simulink model "APID"  (R2021a)
settings: Solver=VariableStepAuto  StartTime=0.0  StopTime=100  RelTol=1e-6  AbsTol=1e-6
undefined symbols (not defined in the file or in its folder): DiscIntNeverNeededParam, G, k, Solar_time, wind, wind_time
libraries: powerlib_extras x24, simulink x2
(part 1 of 2)
settings Model: Creator=hp  LastModifiedBy=hp
settings SolverCC: ZeroCrossAlgorithm=Adaptive
settings DataIOCC: ReturnWorkspaceOutputs=off
settings DebuggingCC: MaskedZcDiagnostic=none  IgnoredZcDiagnostic=none

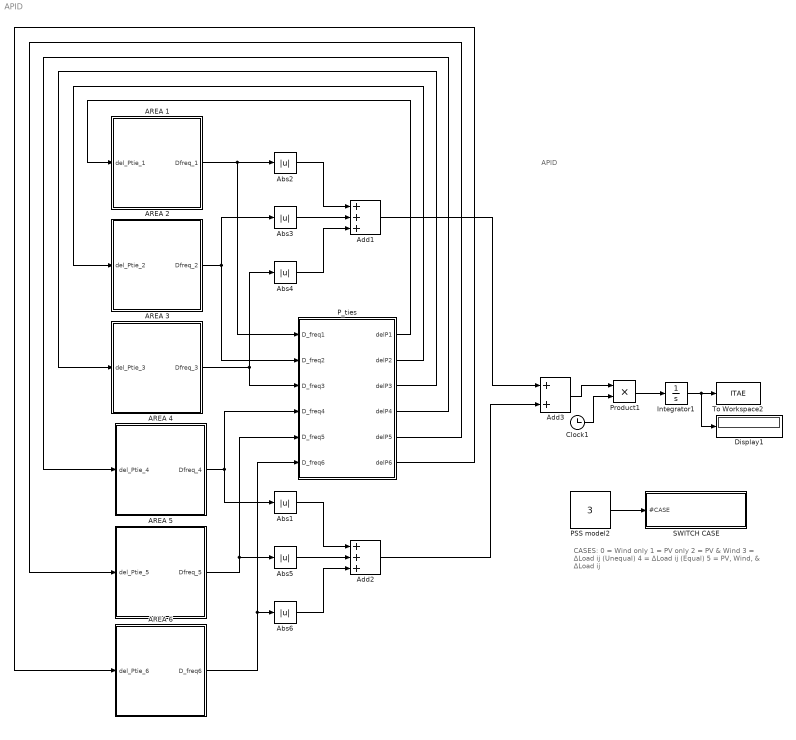
== system APID ==
  note: APID
  note: CASES:
      |
      | 0 = Wind only
      | 1 = PV only
      | 2 = PV & Wind
      | 3 = ΔLoad ij (Unequal)
      | 4 = ΔLoad ij (Equal)
      | 5 = PV, Wind, & ΔLoad ij
  AREA 1 : Subsystem
  AREA 2 : Subsystem
  AREA 3 : Subsystem
  AREA 4 : Subsystem
  AREA 5 : Subsystem
  AREA 6 : Subsystem
  Abs{1..6} (6 alike) : Abs
  Add1 : Sum  Inputs=+++
  Add2 : Sum  Inputs=+++
  Add3 : Sum
  Clock1 : Clock
  Display1 : Display
  Integrator1 : Integrator
  PSS model2 : Constant  Value=3
  P_ties : Subsystem
  Product1 : Product
  SWITCH CASE : Subsystem
  To Workspace2 : ToWorkspace  VariableName=ITAE  SampleTime=-1
      settings: Save2DSignal=2-D array (concatenate along first dimension)
  wires:
  P_ties/1(delP1) -> AREA 1/1(del_Ptie_1)
  Abs2/1 -> Add1/1
  AREA 1/1(Dfreq_1) -> P_ties/1(D_freq1), Abs2/1
  Abs4/1 -> Add1/3
  Abs3/1 -> Add1/2
  P_ties/5(delP5) -> AREA 5/1(del_Ptie_5)
  P_ties/4(delP4) -> AREA 4/1(del_Ptie_4)
  Clock1/1 -> Product1/2
  P_ties/6(delP6) -> AREA 6/1(del_Ptie_6)
  P_ties/2(delP2) -> AREA 2/1(del_Ptie_2)
  AREA 3/1(Dfreq_3) -> P_ties/3(D_freq3), Abs4/1
  Product1/1 -> Integrator1/1
  AREA 2/1("Dfreq_2   ") -> P_ties/2(D_freq2), Abs3/1
  Integrator1/1 -> To Workspace2/1, Display1/1
  P_ties/3(delP3) -> AREA 3/1(del_Ptie_3)
  Abs5/1 -> Add2/2
  Abs6/1 -> Add2/3
  Abs1/1 -> Add2/1
  AREA 4/1(Dfreq_4) -> Abs1/1, P_ties/4(D_freq4)
  AREA 5/1(Dfreq_5) -> P_ties/5(D_freq5), Abs5/1
  AREA 6/1(D_freq6) -> P_ties/6(D_freq6), Abs6/1
  Add3/1 -> Product1/1
  Add1/1 -> Add3/1
  Add2/1 -> Add3/2
  PSS model2/1 -> SWITCH CASE/1(#CASE)

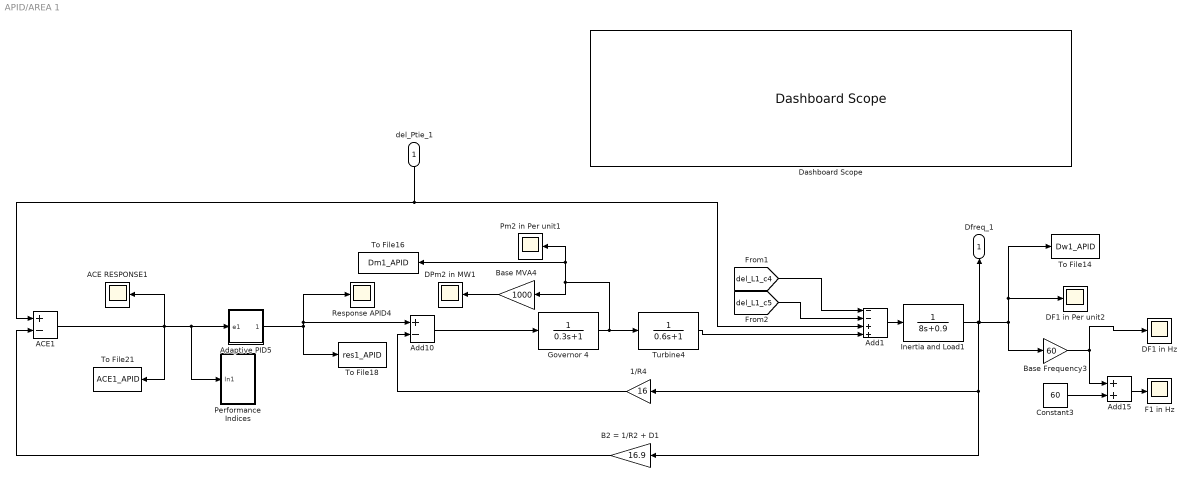
== system APID/AREA 1 ==
  del_Ptie_1 : Inport
  1/R4 : Gain  Gain=16
  ACE RESPONSE1 : Scope
  ACE1 : Sum  Inputs=+-
  Adaptive PID5 : Subsystem  mask{gamma=k}
  Add1 : Sum  Inputs=--++
  Add10 : Sum  Inputs=+-
  Add15 : Sum
  B2 = 1/R2 + D1 : Gain  Gain=16.9
  Base Frequency3 : Gain  Gain=60
  Base MVA4 : Gain  Gain=1000
  Constant3 : Constant  Value=60
  DF1 in Hz : Scope
  DF1 in Per unit2 : Scope
  DPm2 in MW1 : Scope
  Dashboard Scope : DashboardScope
  F1 in Hz : Scope
  Governor 4 : TransferFcn  Denominator=[0.3 1]
  Inertia and Load1 : TransferFcn  Denominator=[8 0.9]
  Performance Indices : Subsystem
  Pm2 in Per unit1 : Scope
  Response APID4 : Scope
  To File14 : ToFile  Filename=Dw1_APID  MatrixName=Dw1_APID
  To File16 : ToFile  Filename=Dm1_APID  MatrixName=Dm1_APID
  To File18 : ToFile  Filename=res1_APID  MatrixName=res1_APID
  To File21 : ToFile  Filename=ACE1_APID  MatrixName=ACE1_APID
  Turbine4 : TransferFcn  Denominator=[0.6 1]
  Dfreq_1 : Outport
  wires:
  Base Frequency3/1 -> DF1 in Hz/1, Add15/1
  Add1/1 -> Inertia and Load1/1
  1/R4/1 -> Add10/2
  Add15/1 -> F1 in Hz/1
  B2 = 1/R2 + D1/1 -> ACE1/2
  Governor 4/1 -> To File16/1, Pm2 in Per unit1/1, Base MVA4/1, Turbine4/1
  Inertia and Load1/1 -> Base Frequency3/1, To File14/1, DF1 in Per unit2/1, Dfreq_1/1, 1/R4/1, B2 = 1/R2 + D1/1
  Base MVA4/1 -> DPm2 in MW1/1
  ACE1/1 -> Adaptive PID5/1(e1), Performance Indices/1(In1), To File21/1, ACE RESPONSE1/1
  Adaptive PID5/1(u(t)) -> Response APID4/1, Add10/1, To File18/1
  Constant3/1 -> Add15/2
  Add10/1 -> Governor 4/1
  [del_L1_c5] -> Add1/2
  Turbine4/1 -> Add1/4
  del_Ptie_1/1 -> ACE1/1, Add1/3
  [del_L1_c4] -> Add1/1

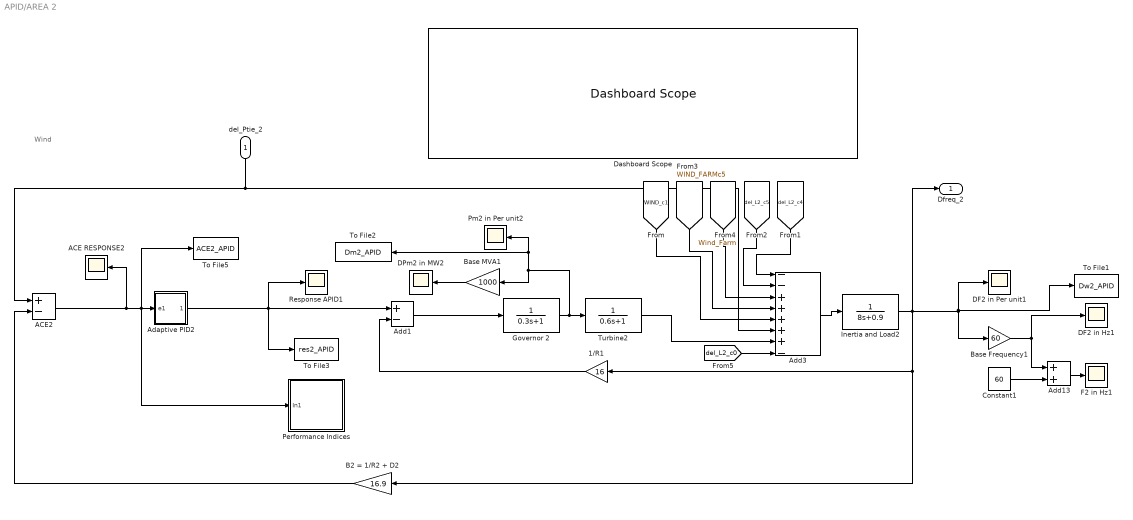
== system APID/AREA 2 ==
  note: Wind
  del_Ptie_2 : Inport
  1/R1 : Gain  Gain=16
  ACE RESPONSE2 : Scope
  ACE2 : Sum  Inputs=+-
  Adaptive PID2 : Subsystem  mask{gamma=k}
  Add1 : Sum  Inputs=+-
  Add13 : Sum
  Add3 : Sum  Inputs=--+++++-
  B2 = 1/R2 + D2 : Gain  Gain=16.9
  Base Frequency1 : Gain  Gain=60
  Base MVA1 : Gain  Gain=1000
  Constant1 : Constant  Value=60
  DF2 in Hz1 : Scope
  DF2 in Per unit1 : Scope
  DPm2 in MW2 : Scope
  Dashboard Scope : DashboardScope
  F2 in Hz1 : Scope
  Governor 2 : TransferFcn  Denominator=[0.3 1]
  Inertia and Load2 : TransferFcn  Denominator=[8 0.9]
  Performance Indices : Subsystem
  Pm2 in Per unit2 : Scope
  Response APID1 : Scope
  To File1 : ToFile  Filename=Dw2_APID  MatrixName=Dw2_APID
  To File2 : ToFile  Filename=Dm2_APID  MatrixName=Dm2_APID
  To File3 : ToFile  Filename=res2_APID  MatrixName=res2_APID
  To File5 : ToFile  Filename=ACE2_APID  MatrixName=ACE2_APID
  Turbine2 : TransferFcn  Denominator=[0.6 1]
  "Dfreq_2   " : Outport
  wires:
  Add13/1 -> F2 in Hz1/1
  1/R1/1 -> Add1/2
  Base Frequency1/1 -> Add13/1, DF2 in Hz1/1
  Constant1/1 -> Add13/2
  Governor 2/1 -> Turbine2/1, Base MVA1/1, To File2/1, Pm2 in Per unit2/1
  Add3/1 -> Inertia and Load2/1
  B2 = 1/R2 + D2/1 -> ACE2/2
  Inertia and Load2/1 -> 1/R1/1, B2 = 1/R2 + D2/1, "Dfreq_2   "/1, DF2 in Per unit1/1, To File1/1, Base Frequency1/1
  Base MVA1/1 -> DPm2 in MW2/1
  ACE2/1 -> Performance Indices/1(In1), Adaptive PID2/1(e1), To File5/1, ACE RESPONSE2/1
  Add1/1 -> Governor 2/1
  Adaptive PID2/1(u(t)) -> Add1/1, Response APID1/1, To File3/1
  Turbine2/1 -> Add3/7
  [del_L2_c5] -> Add3/2
  del_Ptie_2/1 -> Add3/6, ACE2/1
  [WIND_FARMc5] -> Add3/4
  [WIND_c1] -> Add3/5
  [Wind_Farm] -> Add3/3
  [del_L2_c4] -> Add3/1
  [del_L2_c0] -> Add3/8

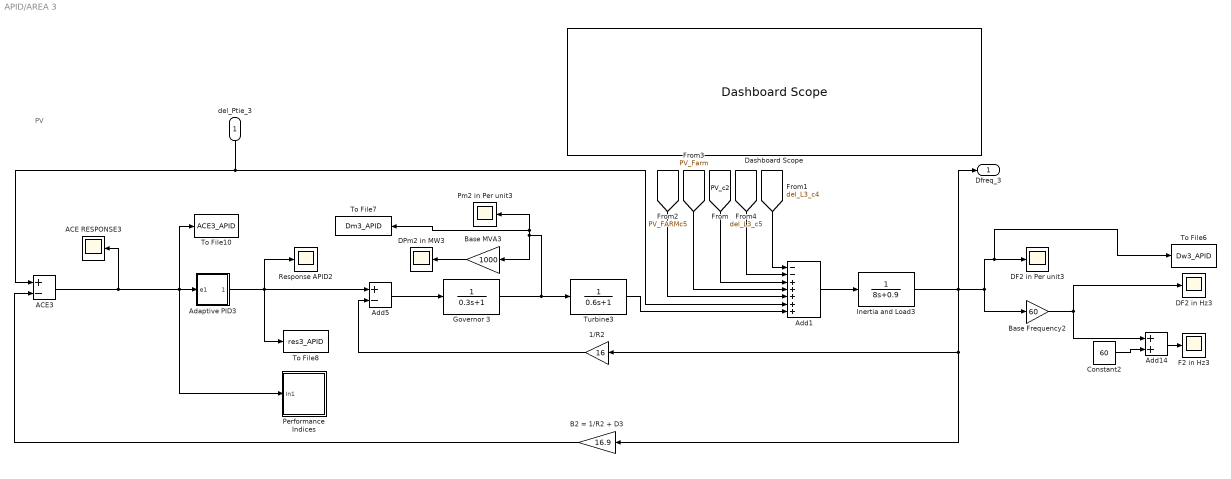
== system APID/AREA 3 ==
  note: PV
  del_Ptie_3 : Inport
  1/R2 : Gain  Gain=16
  ACE RESPONSE3 : Scope
  ACE3 : Sum  Inputs=+-
  Adaptive PID3 : Subsystem  mask{gamma=k}
  Add1 : Sum  Inputs=--+++++
  Add14 : Sum
  Add5 : Sum  Inputs=+-
  B2 = 1/R2 + D3 : Gain  Gain=16.9
  Base Frequency2 : Gain  Gain=60
  Base MVA3 : Gain  Gain=1000
  Constant2 : Constant  Value=60
  DF2 in Hz3 : Scope
  DF2 in Per unit3 : Scope
  DPm2 in MW3 : Scope
  Dashboard Scope : DashboardScope
  F2 in Hz3 : Scope
  Governor 3 : TransferFcn  Denominator=[0.3 1]
  Inertia and Load3 : TransferFcn  Denominator=[8 0.9]
  Performance Indices : Subsystem
  Pm2 in Per unit3 : Scope
  Response APID2 : Scope
  To File10 : ToFile  Filename=ACE3_APID  MatrixName=ACE3_APID
  To File6 : ToFile  Filename=Dw3_APID  MatrixName=Dw3_APID
  To File7 : ToFile  Filename=Dm3_APID  MatrixName=Dm3_APID
  To File8 : ToFile  Filename=res3_APID  MatrixName=res3_APID
  Turbine3 : TransferFcn  Denominator=[0.6 1]
  Dfreq_3 : Outport
  wires:
  Constant2/1 -> Add14/2
  Base MVA3/1 -> DPm2 in MW3/1
  Base Frequency2/1 -> Add14/1, DF2 in Hz3/1
  B2 = 1/R2 + D3/1 -> ACE3/2
  Add1/1 -> Inertia and Load3/1
  Add14/1 -> F2 in Hz3/1
  1/R2/1 -> Add5/2
  Governor 3/1 -> Turbine3/1, Base MVA3/1, To File7/1, Pm2 in Per unit3/1
  ACE3/1 -> Performance Indices/1(In1), To File10/1, Adaptive PID3/1(e1), ACE RESPONSE3/1
  Adaptive PID3/1(u(t)) -> Response APID2/1, Add5/1, To File8/1
  Add5/1 -> Governor 3/1
  Inertia and Load3/1 -> Dfreq_3/1, Base Frequency2/1, To File6/1, DF2 in Per unit3/1, B2 = 1/R2 + D3/1, 1/R2/1
  [PV_FARMc5] -> Add1/5
  Turbine3/1 -> Add1/7
  [del_L3_c5] -> Add1/2
  [del_L3_c4] -> Add1/1
  del_Ptie_3/1 -> Add1/6, ACE3/1
  [PV_c2] -> Add1/3
  [PV_Farm] -> Add1/4

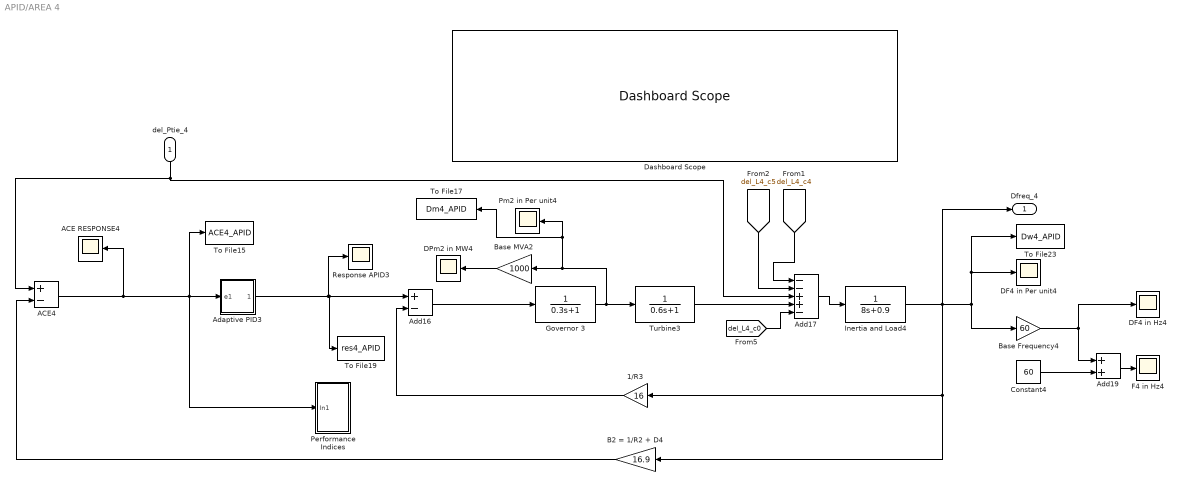
== system APID/AREA 4 ==
  del_Ptie_4 : Inport
  1/R3 : Gain  Gain=16
  ACE RESPONSE4 : Scope
  ACE4 : Sum  Inputs=+-
  Adaptive PID3 : Subsystem  mask{gamma=k}
  Add16 : Sum  Inputs=+-
  Add17 : Sum  Inputs=--++-
  Add19 : Sum
  B2 = 1/R2 + D4 : Gain  Gain=16.9
  Base Frequency4 : Gain  Gain=60
  Base MVA2 : Gain  Gain=1000
  Constant4 : Constant  Value=60
  DF4 in Hz4 : Scope
  DF4 in Per unit4 : Scope
  DPm2 in MW4 : Scope
  Dashboard Scope : DashboardScope
  F4 in Hz4 : Scope
  Governor 3 : TransferFcn  Denominator=[0.3 1]
  Inertia and Load4 : TransferFcn  Denominator=[8 0.9]
  Performance Indices : Subsystem
  Pm2 in Per unit4 : Scope
  Response APID3 : Scope
  To File15 : ToFile  Filename=ACE4_APID  MatrixName=ACE4_APID
  To File17 : ToFile  Filename=Dm4_APID  MatrixName=Dm4_APID
  To File19 : ToFile  Filename=res4_APID  MatrixName=res4_APID
  To File23 : ToFile  Filename=Dw4_APID  MatrixName=Dw4_APID
  Turbine3 : TransferFcn  Denominator=[0.6 1]
  Dfreq_4 : Outport
  wires:
  Add17/1 -> Inertia and Load4/1
  Add19/1 -> F4 in Hz4/1
  Constant4/1 -> Add19/2
  Governor 3/1 -> Turbine3/1, Base MVA2/1, To File17/1, Pm2 in Per unit4/1
  B2 = 1/R2 + D4/1 -> ACE4/2
  1/R3/1 -> Add16/2
  Inertia and Load4/1 -> Dfreq_4/1, To File23/1, DF4 in Per unit4/1, Base Frequency4/1, 1/R3/1, B2 = 1/R2 + D4/1
  Base Frequency4/1 -> Add19/1, DF4 in Hz4/1
  Base MVA2/1 -> DPm2 in MW4/1
  Add16/1 -> Governor 3/1
  ACE4/1 -> Adaptive PID3/1(e1), Performance Indices/1(In1), To File15/1, ACE RESPONSE4/1
  del_Ptie_4/1 -> Add17/3, ACE4/1
  Turbine3/1 -> Add17/4
  Adaptive PID3/1(u(t)) -> Response APID3/1, To File19/1, Add16/1
  [del_L4_c5] -> Add17/2
  [del_L4_c4] -> Add17/1
  [del_L4_c0] -> Add17/5

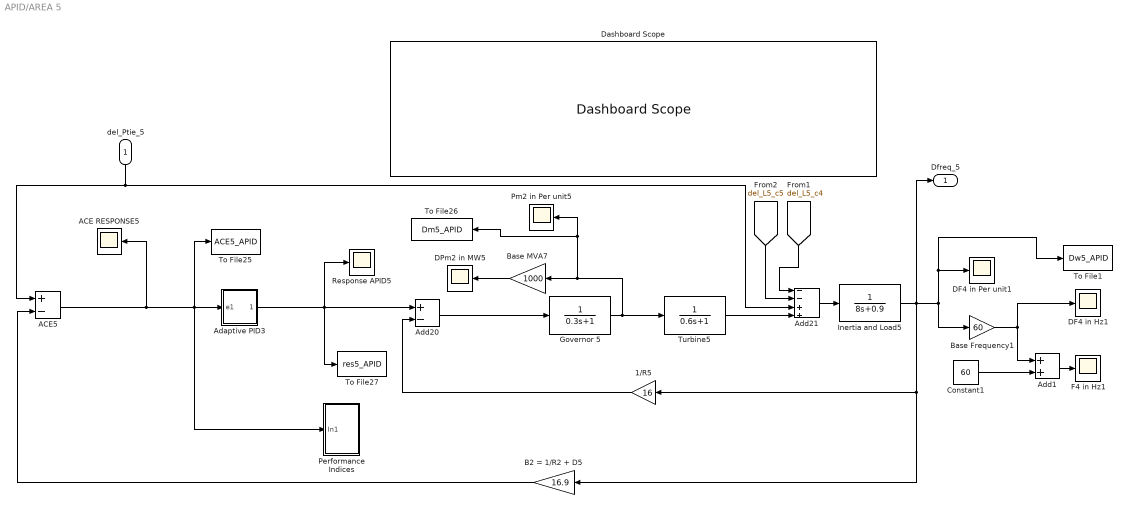
== system APID/AREA 5 ==
  del_Ptie_5 : Inport
  1/R5 : Gain  Gain=16
  ACE RESPONSE5 : Scope
  ACE5 : Sum  Inputs=+-
  Adaptive PID3 : Subsystem  mask{gamma=k}
  Add1 : Sum
  Add20 : Sum  Inputs=+-
  Add21 : Sum  Inputs=--++
  B2 = 1/R2 + D5 : Gain  Gain=16.9
  Base Frequency1 : Gain  Gain=60
  Base MVA7 : Gain  Gain=1000
  Constant1 : Constant  Value=60
  DF4 in Hz1 : Scope
  DF4 in Per unit1 : Scope
  DPm2 in MW5 : Scope
  Dashboard Scope : DashboardScope
  F4 in Hz1 : Scope
  Governor 5 : TransferFcn  Denominator=[0.3 1]
  Inertia and Load5 : TransferFcn  Denominator=[8 0.9]
  Performance Indices : Subsystem
  Pm2 in Per unit5 : Scope
  Response APID5 : Scope
  To File1 : ToFile  Filename=Dw5_APID  MatrixName=Dw5_APID
  To File25 : ToFile  Filename=ACE5_APID  MatrixName=ACE5_APID
  To File26 : ToFile  Filename=Dm5_APID  MatrixName=Dm5_APID
  To File27 : ToFile  Filename=res5_APID  MatrixName=res5_APID
  Turbine5 : TransferFcn  Denominator=[0.6 1]
  Dfreq_5 : Outport
  wires:
  Constant1/1 -> Add1/2
  Add1/1 -> F4 in Hz1/1
  Base Frequency1/1 -> Add1/1, DF4 in Hz1/1
  B2 = 1/R2 + D5/1 -> ACE5/2
  Governor 5/1 -> Turbine5/1, Base MVA7/1, To File26/1, Pm2 in Per unit5/1
  Base MVA7/1 -> DPm2 in MW5/1
  Add21/1 -> Inertia and Load5/1
  1/R5/1 -> Add20/2
  Inertia and Load5/1 -> B2 = 1/R2 + D5/1, 1/R5/1, Dfreq_5/1, Base Frequency1/1, To File1/1, DF4 in Per unit1/1
  ACE5/1 -> Performance Indices/1(In1), Adaptive PID3/1(e1), To File25/1, ACE RESPONSE5/1
  del_Ptie_5/1 -> Add21/3, ACE5/1
  Turbine5/1 -> Add21/4
  Add20/1 -> Governor 5/1
  Adaptive PID3/1(u(t)) -> To File27/1, Response APID5/1, Add20/1
  [del_L5_c5] -> Add21/2
  [del_L5_c4] -> Add21/1

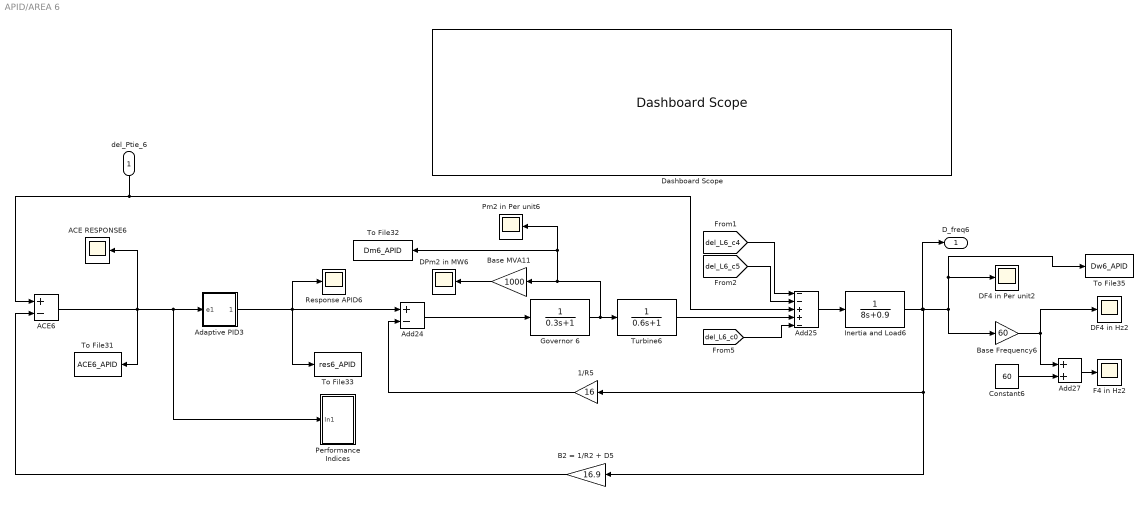
== system APID/AREA 6 ==
  del_Ptie_6 : Inport
  1/R5 : Gain  Gain=16
  ACE RESPONSE6 : Scope
  ACE6 : Sum  Inputs=+-
  Adaptive PID3 : Subsystem  mask{gamma=k}
  Add24 : Sum  Inputs=+-
  Add25 : Sum  Inputs=--++-
  Add27 : Sum
  B2 = 1/R2 + D5 : Gain  Gain=16.9
  Base Frequency6 : Gain  Gain=60
  Base MVA11 : Gain  Gain=1000
  Constant6 : Constant  Value=60
  DF4 in Hz2 : Scope
  DF4 in Per unit2 : Scope
  DPm2 in MW6 : Scope
  Dashboard Scope : DashboardScope
  F4 in Hz2 : Scope
  Governor 6 : TransferFcn  Denominator=[0.3 1]
  Inertia and Load6 : TransferFcn  Denominator=[8 0.9]
  Performance Indices : Subsystem
  Pm2 in Per unit6 : Scope
  Response APID6 : Scope
  To File31 : ToFile  Filename=ACE6_APID  MatrixName=ACE6_APID
  To File32 : ToFile  Filename=Dm6_APID  MatrixName=Dm6_APID
  To File33 : ToFile  Filename=res6_APID  MatrixName=res6_APID
  To File35 : ToFile  Filename=Dw6_APID  MatrixName=Dw6_APID
  Turbine6 : TransferFcn  Denominator=[0.6 1]
  D_freq6 : Outport
  wires:
  Constant6/1 -> Add27/2
  Base Frequency6/1 -> Add27/1, DF4 in Hz2/1
  Base MVA11/1 -> DPm2 in MW6/1
  Add27/1 -> F4 in Hz2/1
  Inertia and Load6/1 -> D_freq6/1, B2 = 1/R2 + D5/1, 1/R5/1, To File35/1, DF4 in Per unit2/1, Base Frequency6/1
  Governor 6/1 -> Turbine6/1, Base MVA11/1, Pm2 in Per unit6/1, To File32/1
  Add25/1 -> Inertia and Load6/1
  ACE6/1 -> To File31/1, Performance Indices/1(In1), Adaptive PID3/1(e1), ACE RESPONSE6/1
  Turbine6/1 -> Add25/4
  Add24/1 -> Governor 6/1
  Adaptive PID3/1(u(t)) -> To File33/1, Response APID6/1, Add24/1
  del_Ptie_6/1 -> Add25/3, ACE6/1
  1/R5/1 -> Add24/2
  B2 = 1/R2 + D5/1 -> ACE6/2
  [del_L6_c5] -> Add25/2
  [del_L6_c4] -> Add25/1
  [del_L6_c0] -> Add25/5

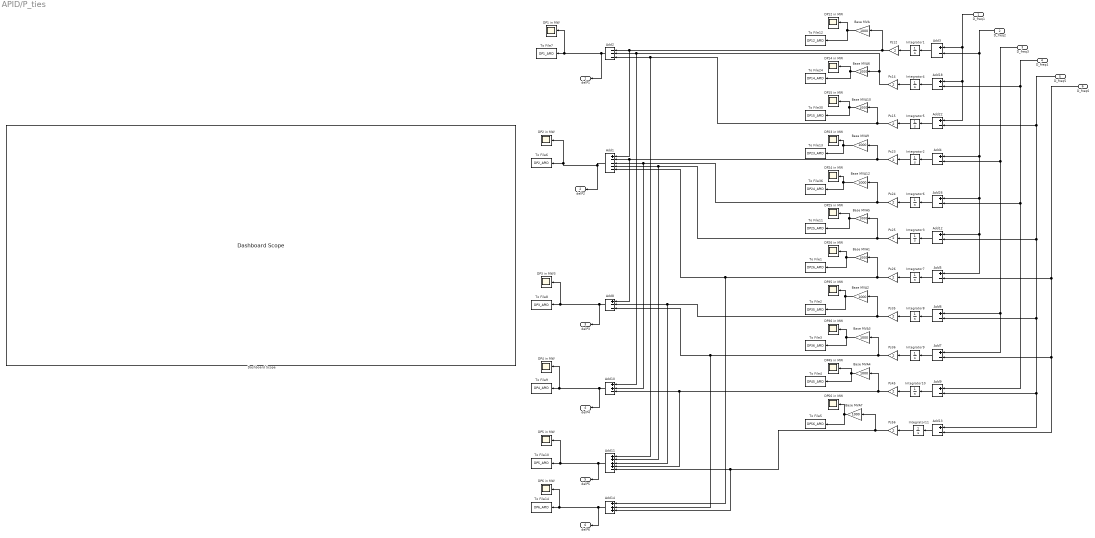
== system APID/P_ties ==
  D_freq1 : Inport
  D_freq2 : Inport  Port=2
  D_freq3 : Inport  Port=3
  D_freq4 : Inport  Port=4
  D_freq5 : Inport  Port=5
  D_freq6 : Inport  Port=6
  Add1 : Sum  Inputs=+----
  Add10 : Sum  Inputs=++-
  Add11 : Sum  Inputs=++++-
  Add{3..7,9,12..13,18,22,26} (11 alike) : Sum  Inputs=+-
  Add14 : Sum  Inputs=+++
  Add2 : Sum  Inputs=---
  Add8 : Sum  Inputs=+--
  Base MVA{,1..7,9..10,12} (11 alike) : Gain  Gain=1000
  DP1 in MW : Scope
  DP12 in MW : Scope
  DP14 in MW : Scope
  DP15 in MW : Scope
  DP2 in MW : Scope
  DP23 in MW : Scope
  DP24 in MW : Scope
  DP25 in MW : Scope
  DP26 in MW : Scope
  DP3 in MW3 : Scope
  DP35 in MW : Scope
  DP36 in MW : Scope
  DP4 in MW : Scope
  DP45 in MW : Scope
  DP5 in MW : Scope
  DP56 in MW : Scope
  DP6 in MW : Scope
  Dashboard Scope : DashboardScope
  Integrator{1..11} (11 alike) : Integrator
  Ps{12,14..15,23..26,35..36,45,56} (11 alike) : Gain  Gain=2
  To File1 : ToFile  Filename=DP26_APID  MatrixName=DP26_APID
  To File10 : ToFile  Filename=DP5_APID  MatrixName=DP5_APID
  To File11 : ToFile  Filename=DP25_APID  MatrixName=DP25_APID
  To File12 : ToFile  Filename=DP12_APID  MatrixName=DP12_APID
  To File13 : ToFile  Filename=DP23_APID  MatrixName=DP23_APID
  To File14 : ToFile  Filename=DP6_APID  MatrixName=DP6_APID
  To File2 : ToFile  Filename=DP35_APID  MatrixName=DP35_APID
  To File24 : ToFile  Filename=DP14_APID  MatrixName=DP14_APID
  To File3 : ToFile  Filename=DP36_APID  MatrixName=DP36_APID
  To File30 : ToFile  Filename=DP15_APID  MatrixName=DP15_APID
  To File36 : ToFile  Filename=DP24_APID  MatrixName=DP24_APID
  To File4 : ToFile  Filename=DP45_APID  MatrixName=DP45_APID
  To File5 : ToFile  Filename=DP56_APID  MatrixName=DP56_APID
  To File6 : ToFile  Filename=DP2_APID  MatrixName=DP2_APID
  To File7 : ToFile  Filename=DP1_APID  MatrixName=DP1_APID
  To File8 : ToFile  Filename=DP3_APID  MatrixName=DP3_APID
  To File9 : ToFile  Filename=DP4_APID  MatrixName=DP4_APID
  delP1 : Outport
  delP2 : Outport  Port=2
  delP3 : Outport  Port=3
  delP4 : Outport  Port=4
  delP5 : Outport  Port=5
  delP6 : Outport  Port=6
  wires:
  Ps12/1 -> Add1/1, Add2/1, Base MVA/1
  Add3/1 -> Integrator1/1
  Integrator1/1 -> Ps12/1
  Base MVA/1 -> To File12/1, DP12 in MW/1
  D_freq1/1 -> Add22/1, Add18/1, Add3/1
  D_freq2/1 -> Add5/1, Add12/1, Add26/1, Add4/1, Add3/2
  Ps14/1 -> Add10/1, Add2/2, Base MVA6/1
  Integrator4/1 -> Ps14/1
  Add18/1 -> Integrator4/1
  Base MVA6/1 -> To File24/1, DP14 in MW/1
  D_freq4/1 -> Add9/1, Add26/2, Add18/2
  Base MVA10/1 -> To File30/1, DP15 in MW/1
  Ps15/1 -> Add11/1, Add2/3, Base MVA10/1
  Integrator5/1 -> Ps15/1
  Add22/1 -> Integrator5/1
  D_freq5/1 -> Add9/2, Add13/1, Add6/2, Add12/2, Add22/2
  Integrator2/1 -> Ps23/1
  Add4/1 -> Integrator2/1
  Ps23/1 -> Base MVA9/1, Add8/1, Add1/2
  Base MVA9/1 -> DP23 in MW/1, To File13/1
  Base MVA12/1 -> DP24 in MW/1, To File36/1
  Integrator6/1 -> Ps24/1
  Ps24/1 -> Add10/2, Add1/3, Base MVA12/1
  Add26/1 -> Integrator6/1
  D_freq3/1 -> Add4/2, Add6/1, Add7/1
  Integrator3/1 -> Ps25/1
  Ps25/1 -> Add11/2, Add1/4, Base MVA5/1
  Base MVA5/1 -> To File11/1, DP25 in MW/1
  Add12/1 -> Integrator3/1
  Add5/1 -> Integrator7/1
  Base MVA1/1 -> To File1/1, DP26 in MW/1
  Integrator7/1 -> Ps26/1
  Ps26/1 -> Add14/1, Add1/5, Base MVA1/1
  D_freq6/1 -> Add5/2, Add7/2, Add13/2
  Base MVA2/1 -> To File2/1, DP35 in MW/1
  Ps35/1 -> Add11/3, Add8/2, Base MVA2/1
  Integrator8/1 -> Ps35/1
  Add6/1 -> Integrator8/1
  Add7/1 -> Integrator9/1
  Base MVA3/1 -> To File3/1, DP36 in MW/1
  Integrator9/1 -> Ps36/1
  Ps36/1 -> Add14/2, Add8/3, Base MVA3/1
  Ps45/1 -> Add11/4, Add10/3, Base MVA4/1
  Add9/1 -> Integrator10/1
  Integrator10/1 -> Ps45/1
  Base MVA4/1 -> DP45 in MW/1, To File4/1
  Integrator11/1 -> Ps56/1
  Add13/1 -> Integrator11/1
  Ps56/1 -> Add14/3, Add11/5, Base MVA7/1
  Base MVA7/1 -> DP56 in MW/1, To File5/1
  Add1/1 -> To File6/1, DP2 in MW/1, delP2/1
  Add2/1 -> DP1 in MW/1, To File7/1, delP1/1
  Add8/1 -> DP3 in MW3/1, To File8/1, delP3/1
  Add10/1 -> DP4 in MW/1, To File9/1, delP4/1
  Add11/1 -> DP5 in MW/1, To File10/1, delP5/1
  Add14/1 -> DP6 in MW/1, To File14/1, delP6/1

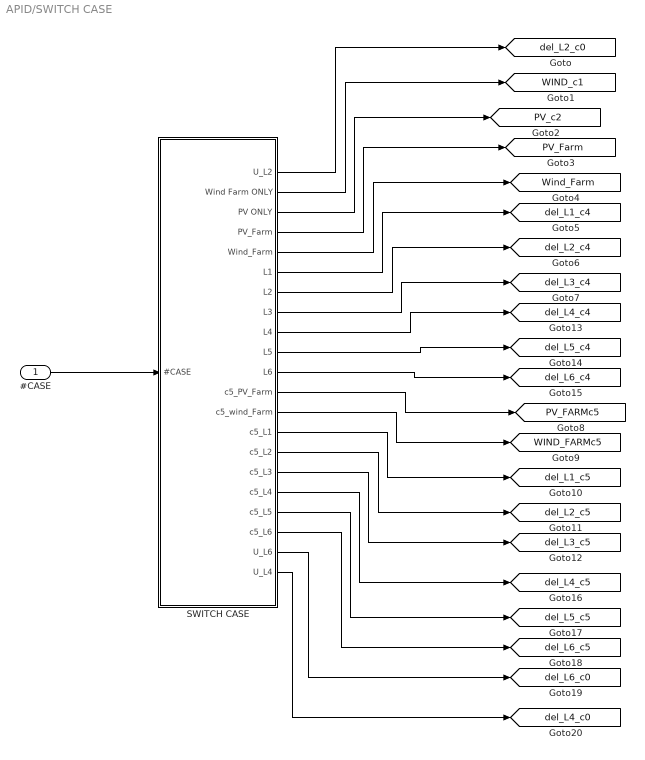
== system APID/SWITCH CASE ==
  #CASE : Inport
  SWITCH CASE : Subsystem
  tag scope: PV_FARMc5=global, PV_Farm=global, PV_c2=global, WIND_FARMc5=global, WIND_c1=global, Wind_Farm=global, del_L1_c4=global, del_L1_c5=global, del_L2_c0=global, del_L2_c4=global, del_L2_c5=global, del_L3_c4=global, del_L3_c5=global, del_L4_c0=global, del_L4_c4=global, del_L4_c5=global, del_L5_c4=global, del_L5_c5=global, del_L6_c0=global, del_L6_c4=global, del_L6_c5=global
  wires:
  SWITCH CASE/9("L4 ") -> [del_L4_c4]
  SWITCH CASE/15(c5_L2) -> [del_L2_c5]
  SWITCH CASE/10("L5 ") -> [del_L5_c4]
  SWITCH CASE/11("L6 ") -> [del_L6_c4]
  SWITCH CASE/1(U_L2) -> [del_L2_c0]
  #CASE/1 -> SWITCH CASE/1(#CASE)
  SWITCH CASE/12(c5_PV_Farm) -> [PV_FARMc5]
  SWITCH CASE/14(c5_L1) -> [del_L1_c5]
  SWITCH CASE/3("PV ONLY ") -> [PV_c2]
  SWITCH CASE/6("L1 ") -> [del_L1_c4]
  SWITCH CASE/4("PV_Farm ") -> [PV_Farm]
  SWITCH CASE/13(c5_wind_Farm) -> [WIND_FARMc5]
  SWITCH CASE/7("L2 ") -> [del_L2_c4]
  SWITCH CASE/2("Wind Farm ONLY ") -> [WIND_c1]
  SWITCH CASE/16("c5_L3 ") -> [del_L3_c5]
  SWITCH CASE/8("L3 ") -> [del_L3_c4]
  SWITCH CASE/5("Wind_Farm ") -> [Wind_Farm]
  SWITCH CASE/17(c5_L4) -> [del_L4_c5]
  SWITCH CASE/18(c5_L5) -> [del_L5_c5]
  SWITCH CASE/19(c5_L6) -> [del_L6_c5]
  SWITCH CASE/20(U_L6) -> [del_L6_c0]
  SWITCH CASE/21(U_L4) -> [del_L4_c0]

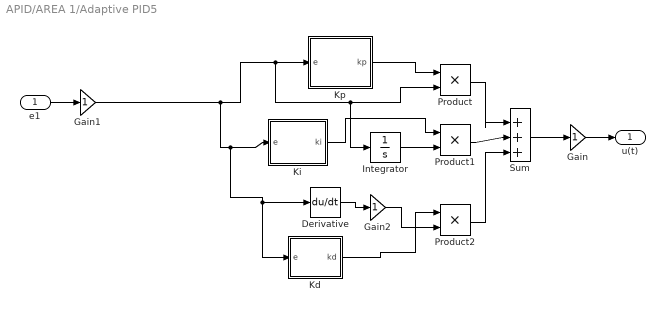
== system APID/AREA 1/Adaptive PID5 ==
  e1 : Inport
  Derivative : Derivative
  Gain : Gain
  Gain1 : Gain
  Gain2 : Gain
  Integrator : Integrator
  Kd : Subsystem
  Ki : Subsystem
  Kp : Subsystem
  Product : Product  RndMeth=Zero
  Product1 : Product  RndMeth=Zero
  Product2 : Product  RndMeth=Zero
  Sum : Sum  Inputs=|+++  SampleTime=0.001
  u(t) : Outport
  wires:
  Gain2/1 -> Product2/2
  Gain1/1 -> Derivative/1, Kd/1(e), Ki/1(e), Integrator/1, Product/2, Kp/1(e)
  Gain/1 -> u(t)/1
  Sum/1 -> Gain/1
  Product2/1 -> Sum/3
  Product1/1 -> Sum/2
  Product/1 -> Sum/1
  Derivative/1 -> Gain2/1
  Integrator/1 -> Product1/2
  e1/1 -> Gain1/1
  Kd/1(kd) -> Product2/1
  Ki/1(ki) -> Product1/1
  Kp/1(kp) -> Product/1

== system APID/AREA 1/Performance Indices ==
  In1 : Inport
  IAE : Subsystem
      mask help:
      | IAE performacne index
      |
      | output = int |input| dt
      mask Display:
      | disp('IAE')
      | port_label('input',1,'e')
      | port_label('output',1,'iae')
  ISE : Subsystem
      mask help:
      | ISE performance index
      |
      | output = int (input)^2 dt
      mask Display:
      | disp('ISE')
      | port_label('input',1,'e')
      | port_label('output',1,'ise')
  ITAE1 : Subsystem
      mask help:
      | ITAE performance index
      |
      | output = int t|input| dt
      mask Display:
      | disp('ITAE')
      | port_label('input',1,'e')
      | port_label('output',1,'itae')
  ITSE : Subsystem
      mask help:
      | ITAE performance index
      |
      | output = int t|input| dt
      mask Display:
      | disp('ITSE')
      | port_label('input',1,'e')
      | port_label('output',1,'itse')
  Subsystem1 : Subsystem
  Subsystem2 : Subsystem
  Subsystem4 : Subsystem
  Subsystem5 : Subsystem
  To File20 : ToFile  Filename=ITAE_ACE_APID_1  MatrixName=ITAE_ACE_APID_1
  To File27 : ToFile  Filename=IAE_ACE_APID_1  MatrixName=IAE_ACE_APID_1
  To File29 : ToFile  Filename=ISE_ACE_APID_1  MatrixName=ISE_ACE_APID_1
  To File30 : ToFile  Filename=ITSE_ACE_APID_1  MatrixName=ITSE_ACE_APID_1
  wires:
  In1/1 -> IAE/1(In1), ISE/1(In1), ITSE/1(In1), ITAE1/1(In1)
  ITAE1/1(Out1) -> Subsystem4/1(In1)
  Subsystem1/1(Out1) -> To File29/1
  Subsystem5/1(Out1) -> To File30/1
  IAE/1(Out1) -> Subsystem2/1(In1)
  Subsystem4/1(DP1) -> To File20/1
  ITSE/1(Out1) -> Subsystem5/1(In1)
  ISE/1(Out1) -> Subsystem1/1(In1)
  Subsystem2/1(Out1) -> To File27/1

== system APID/AREA 2/Adaptive PID2 ==
  e1 : Inport
  Derivative : Derivative
  Gain : Gain
  Gain1 : Gain
  Gain2 : Gain
  Integrator : Integrator
  Kd : Subsystem
  Ki : Subsystem
  Kp : Subsystem
  Product : Product  RndMeth=Zero
  Product1 : Product  RndMeth=Zero
  Product2 : Product  RndMeth=Zero
  Sum : Sum  Inputs=|+++  SampleTime=0.001
  u(t) : Outport
  wires:
  Gain2/1 -> Product2/2
  Gain1/1 -> Derivative/1, Kd/1(e), Ki/1(e), Integrator/1, Product/2, Kp/1(e)
  Gain/1 -> u(t)/1
  Sum/1 -> Gain/1
  Product2/1 -> Sum/3
  Product1/1 -> Sum/2
  Product/1 -> Sum/1
  Derivative/1 -> Gain2/1
  Integrator/1 -> Product1/2
  e1/1 -> Gain1/1
  Kd/1(kd) -> Product2/1
  Ki/1(ki) -> Product1/1
  Kp/1(kp) -> Product/1

== system APID/AREA 2/Performance Indices ==
  In1 : Inport
  IAE : Subsystem
      mask help:
      | IAE performacne index
      |
      | output = int |input| dt
      mask Display:
      | disp('IAE')
      | port_label('input',1,'e')
      | port_label('output',1,'iae')
  ISE : Subsystem
      mask help:
      | ISE performance index
      |
      | output = int (input)^2 dt
      mask Display:
      | disp('ISE')
      | port_label('input',1,'e')
      | port_label('output',1,'ise')
  ITAE1 : Subsystem
      mask help:
      | ITAE performance index
      |
      | output = int t|input| dt
      mask Display:
      | disp('ITAE')
      | port_label('input',1,'e')
      | port_label('output',1,'itae')
  ITSE : Subsystem
      mask help:
      | ITAE performance index
      |
      | output = int t|input| dt
      mask Display:
      | disp('ITSE')
      | port_label('input',1,'e')
      | port_label('output',1,'itse')
  Subsystem1 : Subsystem
  Subsystem2 : Subsystem
  Subsystem3 : Subsystem
  Subsystem5 : Subsystem
  To File27 : ToFile  Filename=IAE_ACE_APID_2  MatrixName=IAE_ACE_APID_2
  To File29 : ToFile  Filename=ISE_ACE_APID_2  MatrixName=ISE_ACE_APID_2
  To File30 : ToFile  Filename=ITSE_ACE_APID_2  MatrixName=ITSE_ACE_APID_2
  To File4 : ToFile  Filename=ITAE_ACE_APID_2  MatrixName=ITAE_ACE_APID_2
  wires:
  ISE/1(Out1) -> Subsystem2/1(In1)
  In1/1 -> IAE/1(In1), ITSE/1(In1), ISE/1(In1), ITAE1/1(In1)
  IAE/1(Out1) -> Subsystem3/1(In1)
  Subsystem1/1(DP1) -> To File4/1
  ITAE1/1(Out1) -> Subsystem1/1(In1)
  ITSE/1(Out1) -> Subsystem5/1(In1)
  Subsystem5/1(Out1) -> To File30/1
  Subsystem2/1(Out1) -> To File29/1
  Subsystem3/1(Out1) -> To File27/1

== system APID/AREA 3/Adaptive PID3 ==
  e1 : Inport
  Derivative : Derivative
  Gain : Gain
  Gain1 : Gain
  Gain2 : Gain
  Integrator : Integrator
  Kd : Subsystem
  Ki : Subsystem
  Kp : Subsystem
  Product : Product  RndMeth=Zero
  Product1 : Product  RndMeth=Zero
  Product2 : Product  RndMeth=Zero
  Sum : Sum  Inputs=|+++  SampleTime=0.001
  u(t) : Outport
  wires:
  Gain2/1 -> Product2/2
  Gain1/1 -> Derivative/1, Kd/1(e), Ki/1(e), Integrator/1, Product/2, Kp/1(e)
  Gain/1 -> u(t)/1
  Sum/1 -> Gain/1
  Product2/1 -> Sum/3
  Product1/1 -> Sum/2
  Product/1 -> Sum/1
  Derivative/1 -> Gain2/1
  Integrator/1 -> Product1/2
  e1/1 -> Gain1/1
  Kd/1(kd) -> Product2/1
  Ki/1(ki) -> Product1/1
  Kp/1(kp) -> Product/1

== system APID/AREA 3/Performance Indices ==
  In1 : Inport
  IAE : Subsystem
      mask help:
      | IAE performacne index
      |
      | output = int |input| dt
      mask Display:
      | disp('IAE')
      | port_label('input',1,'e')
      | port_label('output',1,'iae')
  ISE : Subsystem
      mask help:
      | ISE performance index
      |
      | output = int (input)^2 dt
      mask Display:
      | disp('ISE')
      | port_label('input',1,'e')
      | port_label('output',1,'ise')
  ITAE2 : Subsystem
      mask help:
      | ITAE performance index
      |
      | output = int t|input| dt
      mask Display:
      | disp('ITAE')
      | port_label('input',1,'e')
      | port_label('output',1,'itae')
  ITSE : Subsystem
      mask help:
      | ITAE performance index
      |
      | output = int t|input| dt
      mask Display:
      | disp('ITSE')
      | port_label('input',1,'e')
      | port_label('output',1,'itse')
  Subsystem1 : Subsystem
  Subsystem2 : Subsystem
  Subsystem3 : Subsystem
  Subsystem5 : Subsystem
  To File27 : ToFile  Filename=IAE_ACE_APID_3  MatrixName=IAE_ACE_APID_3
  To File29 : ToFile  Filename=ISE_ACE_APID_3  MatrixName=ISE_ACE_APID_3
  To File30 : ToFile  Filename=ITSE_ACE_APID_3  MatrixName=ITSE_ACE_APID_3
  To File9 : ToFile  Filename=ITAE_ACE_APID_3  MatrixName=ITAE_ACE_APID_3
  wires:
  Subsystem5/1(Out1) -> To File30/1
  IAE/1(Out1) -> Subsystem3/1(In1)
  ITAE2/1(Out1) -> Subsystem2/1(In1)
  ISE/1(Out1) -> Subsystem1/1(In1)
  In1/1 -> IAE/1(In1), ITSE/1(In1), ISE/1(In1), ITAE2/1(In1)
  Subsystem2/1(DP1) -> To File9/1
  Subsystem1/1(Out1) -> To File29/1
  Subsystem3/1(Out1) -> To File27/1
  ITSE/1(Out1) -> Subsystem5/1(In1)

== system APID/AREA 4/Adaptive PID3 ==
  e1 : Inport
  Derivative : Derivative
  Gain : Gain
  Gain1 : Gain
  Gain2 : Gain
  Integrator : Integrator
  Kd : Subsystem
  Ki : Subsystem
  Kp : Subsystem
  Product : Product  RndMeth=Zero
  Product1 : Product  RndMeth=Zero
  Product2 : Product  RndMeth=Zero
  Sum : Sum  Inputs=|+++  SampleTime=0.001
  u(t) : Outport
  wires:
  Gain2/1 -> Product2/2
  Gain1/1 -> Derivative/1, Kd/1(e), Ki/1(e), Integrator/1, Product/2, Kp/1(e)
  Gain/1 -> u(t)/1
  Sum/1 -> Gain/1
  Product2/1 -> Sum/3
  Product1/1 -> Sum/2
  Product/1 -> Sum/1
  Derivative/1 -> Gain2/1
  Integrator/1 -> Product1/2
  e1/1 -> Gain1/1
  Kd/1(kd) -> Product2/1
  Ki/1(ki) -> Product1/1
  Kp/1(kp) -> Product/1

== system APID/AREA 4/Performance Indices ==
  In1 : Inport
  IAE : Subsystem
      mask help:
      | IAE performacne index
      |
      | output = int |input| dt
      mask Display:
      | disp('IAE')
      | port_label('input',1,'e')
      | port_label('output',1,'iae')
  ISE : Subsystem
      mask help:
      | ISE performance index
      |
      | output = int (input)^2 dt
      mask Display:
      | disp('ISE')
      | port_label('input',1,'e')
      | port_label('output',1,'ise')
  ITAE4 : Subsystem
      mask help:
      | ITAE performance index
      |
      | output = int t|input| dt
      mask Display:
      | disp('ITAE')
      | port_label('input',1,'e')
      | port_label('output',1,'itae')
  ITSE : Subsystem
      mask help:
      | ITAE performance index
      |
      | output = int t|input| dt
      mask Display:
      | disp('ITSE')
      | port_label('input',1,'e')
      | port_label('output',1,'itse')
  Subsystem1 : Subsystem
  Subsystem2 : Subsystem
  Subsystem3 : Subsystem
  Subsystem5 : Subsystem
  To File22 : ToFile  Filename=ITAE_ACE_APID_4  MatrixName=ITAE_ACE_APID_4
  To File27 : ToFile  Filename=IAE_ACE_APID_4  MatrixName=IAE_ACE_APID_4
  To File29 : ToFile  Filename=ISE_ACE_APID_4  MatrixName=ISE_ACE_APID_4
  To File30 : ToFile  Filename=ITSE_ACE_APID_4  MatrixName=ITSE_ACE_APID_4
  wires:
  ITSE/1(Out1) -> Subsystem5/1(In1)
  IAE/1(Out1) -> Subsystem2/1(In1)
  ISE/1(Out1) -> Subsystem1/1(In1)
  Subsystem2/1(Out1) -> To File27/1
  Subsystem1/1(Out1) -> To File29/1
  ITAE4/1(Out1) -> Subsystem3/1(In1)
  In1/1 -> IAE/1(In1), ITSE/1(In1), ISE/1(In1), ITAE4/1(In1)
  Subsystem3/1(DP1) -> To File22/1
  Subsystem5/1(Out1) -> To File30/1

== system APID/AREA 5/Adaptive PID3 ==
  e1 : Inport
  Derivative : Derivative
  Gain : Gain
  Gain1 : Gain
  Gain2 : Gain
  Integrator : Integrator
  Kd : Subsystem
  Ki : Subsystem
  Kp : Subsystem
  Product : Product  RndMeth=Zero
  Product1 : Product  RndMeth=Zero
  Product2 : Product  RndMeth=Zero
  Sum : Sum  Inputs=|+++  SampleTime=0.001
  u(t) : Outport
  wires:
  Gain2/1 -> Product2/2
  Gain1/1 -> Derivative/1, Kd/1(e), Ki/1(e), Integrator/1, Product/2, Kp/1(e)
  Gain/1 -> u(t)/1
  Sum/1 -> Gain/1
  Product2/1 -> Sum/3
  Product1/1 -> Sum/2
  Product/1 -> Sum/1
  Derivative/1 -> Gain2/1
  Integrator/1 -> Product1/2
  e1/1 -> Gain1/1
  Kd/1(kd) -> Product2/1
  Ki/1(ki) -> Product1/1
  Kp/1(kp) -> Product/1

== system APID/AREA 5/Performance Indices ==
  In1 : Inport
  IAE : Subsystem
      mask help:
      | IAE performacne index
      |
      | output = int |input| dt
      mask Display:
      | disp('IAE')
      | port_label('input',1,'e')
      | port_label('output',1,'iae')
  ISE : Subsystem
      mask help:
      | ISE performance index
      |
      | output = int (input)^2 dt
      mask Display:
      | disp('ISE')
      | port_label('input',1,'e')
      | port_label('output',1,'ise')
  ITAE5 : Subsystem
      mask help:
      | ITAE performance index
      |
      | output = int t|input| dt
      mask Display:
      | disp('ITAE')
      | port_label('input',1,'e')
      | port_label('output',1,'itae')
  ITSE : Subsystem
      mask help:
      | ITAE performance index
      |
      | output = int t|input| dt
      mask Display:
      | disp('ITSE')
      | port_label('input',1,'e')
      | port_label('output',1,'itse')
  Subsystem1 : Subsystem
  Subsystem2 : Subsystem
  Subsystem3 : Subsystem
  Subsystem5 : Subsystem
  To File2 : ToFile  Filename=IAE_ACE_APID_5  MatrixName=IAE_ACE_APID_5
  To File28 : ToFile  Filename=ITAE_ACE_APID_5  MatrixName=ITAE_ACE_APID_5
  To File29 : ToFile  Filename=ISE_ACE_APID_5  MatrixName=ISE_ACE_APID_5
  To File30 : ToFile  Filename=ITSE_ACE_APID_5  MatrixName=ITSE_ACE_APID_5
  wires:
  In1/1 -> IAE/1(In1), ITSE/1(In1), ISE/1(In1), ITAE5/1(In1)
  ISE/1(Out1) -> Subsystem1/1(In1)
  Subsystem2/1(Out1) -> To File2/1
  Subsystem1/1(Out1) -> To File29/1
  ITAE5/1(Out1) -> Subsystem5/1(In1)
  Subsystem3/1(Out1) -> To File30/1
  IAE/1(Out1) -> Subsystem2/1(In1)
  ITSE/1(Out1) -> Subsystem3/1(In1)
  Subsystem5/1(DP1) -> To File28/1

== system APID/AREA 6/Adaptive PID3 ==
  e1 : Inport
  Derivative : Derivative
  Gain : Gain
  Gain1 : Gain
  Gain2 : Gain
  Integrator : Integrator
  Kd : Subsystem
  Ki : Subsystem
  Kp : Subsystem
  Product : Product  RndMeth=Zero
  Product1 : Product  RndMeth=Zero
  Product2 : Product  RndMeth=Zero
  Sum : Sum  Inputs=|+++  SampleTime=0.001
  u(t) : Outport
  wires:
  Gain2/1 -> Product2/2
  Gain1/1 -> Derivative/1, Kd/1(e), Ki/1(e), Integrator/1, Product/2, Kp/1(e)
  Gain/1 -> u(t)/1
  Sum/1 -> Gain/1
  Product2/1 -> Sum/3
  Product1/1 -> Sum/2
  Product/1 -> Sum/1
  Derivative/1 -> Gain2/1
  Integrator/1 -> Product1/2
  e1/1 -> Gain1/1
  Kd/1(kd) -> Product2/1
  Ki/1(ki) -> Product1/1
  Kp/1(kp) -> Product/1

== system APID/AREA 6/Performance Indices ==
  In1 : Inport
  IAE : Subsystem
      mask help:
      | IAE performacne index
      |
      | output = int |input| dt
      mask Display:
      | disp('IAE')
      | port_label('input',1,'e')
      | port_label('output',1,'iae')
  ISE : Subsystem
      mask help:
      | ISE performance index
      |
      | output = int (input)^2 dt
      mask Display:
      | disp('ISE')
      | port_label('input',1,'e')
      | port_label('output',1,'ise')
  ITAE6 : Subsystem
      mask help:
      | ITAE performance index
      |
      | output = int t|input| dt
      mask Display:
      | disp('ITAE')
      | port_label('input',1,'e')
      | port_label('output',1,'itae')
  ITSE : Subsystem
      mask help:
      | ITAE performance index
      |
      | output = int t|input| dt
      mask Display:
      | disp('ITSE')
      | port_label('input',1,'e')
      | port_label('output',1,'itse')
  Subsystem1 : Subsystem
  Subsystem2 : Subsystem
  Subsystem5 : Subsystem
  Subsystem6 : Subsystem
  To File27 : ToFile  Filename=IAE_ACE_APID_6  MatrixName=IAE_ACE_APID_6
  To File29 : ToFile  Filename=ISE_ACE_APID_6  MatrixName=ISE_ACE_APID_6
  To File30 : ToFile  Filename=ITSE_ACE_APID_6  MatrixName=ITSE_ACE_APID_6
  To File34 : ToFile  Filename=ITAE_ACE_APID_6  MatrixName=ITAE_ACE_APID_6
  wires:
  ISE/1(Out1) -> Subsystem1/1(In1)
  ITAE6/1(Out1) -> Subsystem6/1(In1)
  In1/1 -> IAE/1(In1), ITSE/1(In1), ISE/1(In1), ITAE6/1(In1)
  Subsystem5/1(Out1) -> To File30/1
  Subsystem1/1(Out1) -> To File29/1
  Subsystem6/1(DP1) -> To File34/1
  ITSE/1(Out1) -> Subsystem5/1(In1)
  IAE/1(Out1) -> Subsystem2/1(In1)
  Subsystem2/1(Out1) -> To File27/1

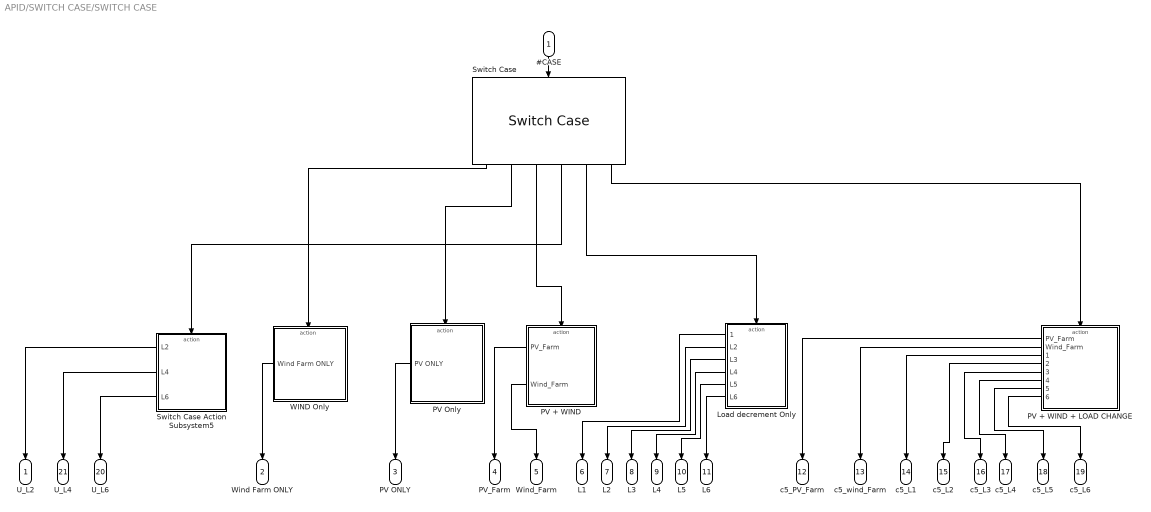
== system APID/SWITCH CASE/SWITCH CASE ==
  #CASE : Inport
  Load decrement Only : Subsystem  TreatAsAtomicUnit=on
  "PV + WIND " : Subsystem  TreatAsAtomicUnit=on
  PV + WIND + LOAD CHANGE : Subsystem  TreatAsAtomicUnit=on
  PV Only : Subsystem  TreatAsAtomicUnit=on
  Switch Case : SwitchCase  CaseConditions={0,1,2,3,4,5}  ShowDefaultCase=off
  Switch Case Action Subsystem5 : Subsystem  TreatAsAtomicUnit=on
  WIND Only : Subsystem  TreatAsAtomicUnit=on
  U_L2 : Outport
  "Wind Farm ONLY " : Outport  Port=2
  "PV ONLY " : Outport  Port=3
  "PV_Farm " : Outport  Port=4
  "Wind_Farm " : Outport  Port=5
  "L1 " : Outport  Port=6
  "L2 " : Outport  Port=7
  "L3 " : Outport  Port=8
  "L4 " : Outport  Port=9
  "L5 " : Outport  Port=10
  "L6 " : Outport  Port=11
  c5_PV_Farm : Outport  Port=12
  c5_wind_Farm : Outport  Port=13
  c5_L1 : Outport  Port=14
  c5_L2 : Outport  Port=15
  "c5_L3 " : Outport  Port=16
  c5_L4 : Outport  Port=17
  c5_L5 : Outport  Port=18
  c5_L6 : Outport  Port=19
  U_L6 : Outport  Port=20
  U_L4 : Outport  Port=21
  wires:
  PV + WIND + LOAD CHANGE/4("2 ") -> c5_L2/1
  PV + WIND + LOAD CHANGE/5("3 ") -> "c5_L3 "/1
  PV + WIND + LOAD CHANGE/2("Wind_Farm ") -> c5_wind_Farm/1
  PV + WIND + LOAD CHANGE/1("PV_Farm ") -> c5_PV_Farm/1
  PV + WIND + LOAD CHANGE/3("1 ") -> c5_L1/1
  #CASE/1 -> Switch Case/1
  "PV + WIND "/2("Wind_Farm ") -> "Wind_Farm "/1
  "PV + WIND "/1("PV_Farm ") -> "PV_Farm "/1
  PV Only/1("PV ONLY ") -> "PV ONLY "/1
  WIND Only/1("Wind Farm ONLY ") -> "Wind Farm ONLY "/1
  Switch Case/5 -> Load decrement Only/Action
  Switch Case/6 -> PV + WIND + LOAD CHANGE/Action
  Load decrement Only/1(" ") -> "L1 "/1
  Load decrement Only/2("L2 ") -> "L2 "/1
  Load decrement Only/3("L3 ") -> "L3 "/1
  Load decrement Only/4("L4 ") -> "L4 "/1
  Load decrement Only/5("L5 ") -> "L5 "/1
  Load decrement Only/6("L6 ") -> "L6 "/1
  PV + WIND + LOAD CHANGE/6(4) -> c5_L4/1
  PV + WIND + LOAD CHANGE/7("5 ") -> c5_L5/1
  PV + WIND + LOAD CHANGE/8("6 ") -> c5_L6/1
  Switch Case Action Subsystem5/1("L2 ") -> U_L2/1
  Switch Case Action Subsystem5/2("L4 ") -> U_L4/1
  Switch Case Action Subsystem5/3("L6 ") -> U_L6/1
  Switch Case/4 -> Switch Case Action Subsystem5/Action
  Switch Case/3 -> "PV + WIND "/Action
  Switch Case/1 -> WIND Only/Action
  Switch Case/2 -> PV Only/Action

== system APID/AREA 1/Adaptive PID5/Kd ==
  e : Inport
  Derivative : Derivative
  Product : Product  Inputs=3  RndMeth=Zero
  Sum2 : Sum
  Unit Delay : UnitDelay  InitialCondition=1.875  SampleTime=-1  HasFrameUpgradeWarning=on
  gamma : Constant  Value=gamma  SampleTime=0.001
  kd : Outport
  wires:
  Derivative/1 -> Product/2
  e/1 -> Product/3, Derivative/1
  gamma/1 -> Product/1
  Unit Delay/1 -> Sum2/1, kd/1
  Sum2/1 -> Unit Delay/1
  Product/1 -> Sum2/2

== system APID/AREA 1/Adaptive PID5/Ki ==
  e : Inport
  Math Function : Math  Operator=square  SignedPower=on  SaturateOnIntegerOverflow=on
  Product1 : Product  Inputs=3  RndMeth=Zero
  Sum1 : Sum
  Unit Delay1 : UnitDelay  InitialCondition=1.875  SampleTime=-1  HasFrameUpgradeWarning=on
  gamma1 : Constant  Value=gamma/2  SampleTime=0.001
  ki : Outport
  wires:
  gamma1/1 -> Product1/3
  Math Function/1 -> Product1/1
  Product1/1 -> Sum1/2
  e/1 -> Product1/2, Math Function/1
  Unit Delay1/1 -> ki/1, Sum1/1
  Sum1/1 -> Unit Delay1/1

== system APID/AREA 1/Adaptive PID5/Kp ==
  e : Inport
  Math Function : Math  Operator=square  SignedPower=on  SaturateOnIntegerOverflow=on
  Product : Product  RndMeth=Zero
  Sum2 : Sum
  Unit Delay : UnitDelay  InitialCondition=1.875  SampleTime=-1  HasFrameUpgradeWarning=on
  gamma : Constant  Value=gamma  SampleTime=0.001
  kp : Outport
  wires:
  Unit Delay/1 -> Sum2/1, kp/1
  Sum2/1 -> Unit Delay/1
  Product/1 -> Sum2/2
  gamma/1 -> Product/2
  Math Function/1 -> Product/1
  e/1 -> Math Function/1

== system APID/AREA 1/Performance Indices/IAE ==
  In1 : Inport
  Abs : Abs
  Discrete-Time Integrator : DiscreteIntegrator  gainval=1  SampleTime=-1  ICPrevOutput=DiscIntNeverNeededParam  ICPrevScaledInput=DiscIntNeverNeededParam
  Out1 : Outport
  wires:
  Abs/1 -> Discrete-Time Integrator/1
  Discrete-Time Integrator/1 -> Out1/1
  In1/1 -> Abs/1

== system APID/AREA 1/Performance Indices/ISE ==
  In1 : Inport
  Discrete-Time Integrator : DiscreteIntegrator  gainval=1  SampleTime=-1  ICPrevOutput=DiscIntNeverNeededParam  ICPrevScaledInput=DiscIntNeverNeededParam
  Math Function : Math  Operator=square  SignedPower=on  SaturateOnIntegerOverflow=on
  Out1 : Outport
  wires:
  In1/1 -> Math Function/1
  Discrete-Time Integrator/1 -> Out1/1
  Math Function/1 -> Discrete-Time Integrator/1

== system APID/AREA 1/Performance Indices/ITAE1 ==
  In1 : Inport
  Abs : Abs
  Clock : Clock
      settings: Decimation=25
  Discrete-Time Integrator : DiscreteIntegrator  gainval=1  SampleTime=-1  ICPrevOutput=DiscIntNeverNeededParam  ICPrevScaledInput=DiscIntNeverNeededParam
  Divide : Product  Inputs=**
  Out1 : Outport
  wires:
  Clock/1 -> Divide/2
  Abs/1 -> Divide/1
  Divide/1 -> Discrete-Time Integrator/1
  In1/1 -> Abs/1
  Discrete-Time Integrator/1 -> Out1/1

== system APID/AREA 1/Performance Indices/ITSE ==
  In1 : Inport
  Clock : Clock
  Discrete-Time Integrator : DiscreteIntegrator  gainval=1  SampleTime=-1  ICPrevOutput=DiscIntNeverNeededParam  ICPrevScaledInput=DiscIntNeverNeededParam
  Divide : Product  Inputs=**
  Math Function : Math  Operator=square  SignedPower=on  SaturateOnIntegerOverflow=on
  Out1 : Outport
  wires:
  Discrete-Time Integrator/1 -> Out1/1
  In1/1 -> Math Function/1
  Divide/1 -> Discrete-Time Integrator/1
  Math Function/1 -> Divide/1
  Clock/1 -> Divide/2

== system APID/AREA 1/Performance Indices/Subsystem1 ==
  In1 : Inport
  Id_ref step : powerlib_extras/Control  Blocks/Timer  t=[0 1]  e=[0 1]
      settings: SourceProductBaseCode=PS
  Prod : Product  InputSameDT=on  SaturateOnIntegerOverflow=on  OutDataTypeStr=Inherit: Same as first input
  Out1 : Outport
  wires:
  Id_ref step/1 -> Prod/2
  In1/1 -> Prod/1
  Prod/1 -> Out1/1

== system APID/AREA 1/Performance Indices/Subsystem2 ==
  In1 : Inport
  Id_ref step : powerlib_extras/Control  Blocks/Timer  t=[0 1]  e=[0 1]
      settings: SourceProductBaseCode=PS
  Prod : Product  InputSameDT=on  SaturateOnIntegerOverflow=on  OutDataTypeStr=Inherit: Same as first input
  Out1 : Outport
  wires:
  Prod/1 -> Out1/1
  In1/1 -> Prod/1
  Id_ref step/1 -> Prod/2

== system APID/AREA 1/Performance Indices/Subsystem4 ==
  In1 : Inport
  Id_ref step : powerlib_extras/Control  Blocks/Timer  t=[0 1]  e=[0 1]
      settings: SourceProductBaseCode=PS
  Prod : Product  InputSameDT=on  SaturateOnIntegerOverflow=on  OutDataTypeStr=Inherit: Same as first input
  DP1 : Outport
  wires:
  Id_ref step/1 -> Prod/2
  In1/1 -> Prod/1
  Prod/1 -> DP1/1

== system APID/AREA 1/Performance Indices/Subsystem5 ==
  In1 : Inport
  Id_ref step : powerlib_extras/Control  Blocks/Timer  t=[0 1]  e=[0 1]
      settings: SourceProductBaseCode=PS
  Prod : Product  InputSameDT=on  SaturateOnIntegerOverflow=on  OutDataTypeStr=Inherit: Same as first input
  Out1 : Outport
  wires:
  Prod/1 -> Out1/1
  In1/1 -> Prod/1
  Id_ref step/1 -> Prod/2

== system APID/AREA 2/Adaptive PID2/Kd ==
  e : Inport
  Derivative : Derivative
  Product : Product  Inputs=3  RndMeth=Zero
  Sum2 : Sum
  Unit Delay : UnitDelay  InitialCondition=1.875  SampleTime=-1  HasFrameUpgradeWarning=on
  gamma : Constant  Value=gamma  SampleTime=0.001
  kd : Outport
  wires:
  Derivative/1 -> Product/2
  e/1 -> Product/3, Derivative/1
  gamma/1 -> Product/1
  Unit Delay/1 -> Sum2/1, kd/1
  Sum2/1 -> Unit Delay/1
  Product/1 -> Sum2/2

== system APID/AREA 2/Adaptive PID2/Ki ==
  e : Inport
  Math Function : Math  Operator=square  SignedPower=on  SaturateOnIntegerOverflow=on
  Product1 : Product  Inputs=3  RndMeth=Zero
  Sum1 : Sum
  Unit Delay1 : UnitDelay  InitialCondition=1.875  SampleTime=-1  HasFrameUpgradeWarning=on
  gamma1 : Constant  Value=gamma/2  SampleTime=0.001
  ki : Outport
  wires:
  gamma1/1 -> Product1/3
  Math Function/1 -> Product1/1
  Product1/1 -> Sum1/2
  e/1 -> Product1/2, Math Function/1
  Unit Delay1/1 -> ki/1, Sum1/1
  Sum1/1 -> Unit Delay1/1

== system APID/AREA 2/Adaptive PID2/Kp ==
  e : Inport
  Math Function : Math  Operator=square  SignedPower=on  SaturateOnIntegerOverflow=on
  Product : Product  RndMeth=Zero
  Sum2 : Sum
  Unit Delay : UnitDelay  InitialCondition=1.875  SampleTime=-1  HasFrameUpgradeWarning=on
  gamma : Constant  Value=gamma  SampleTime=0.001
  kp : Outport
  wires:
  Unit Delay/1 -> Sum2/1, kp/1
  Sum2/1 -> Unit Delay/1
  Product/1 -> Sum2/2
  gamma/1 -> Product/2
  Math Function/1 -> Product/1
  e/1 -> Math Function/1

== system APID/AREA 2/Performance Indices/IAE ==
  In1 : Inport
  Abs : Abs
  Discrete-Time Integrator : DiscreteIntegrator  gainval=1  SampleTime=-1  ICPrevOutput=DiscIntNeverNeededParam  ICPrevScaledInput=DiscIntNeverNeededParam
  Out1 : Outport
  wires:
  Abs/1 -> Discrete-Time Integrator/1
  Discrete-Time Integrator/1 -> Out1/1
  In1/1 -> Abs/1

== system APID/AREA 2/Performance Indices/ISE ==
  In1 : Inport
  Discrete-Time Integrator : DiscreteIntegrator  gainval=1  SampleTime=-1  ICPrevOutput=DiscIntNeverNeededParam  ICPrevScaledInput=DiscIntNeverNeededParam
  Math Function : Math  Operator=square  SignedPower=on  SaturateOnIntegerOverflow=on
  Out1 : Outport
  wires:
  In1/1 -> Math Function/1
  Discrete-Time Integrator/1 -> Out1/1
  Math Function/1 -> Discrete-Time Integrator/1

== system APID/AREA 2/Performance Indices/ITAE1 ==
  In1 : Inport
  Abs : Abs
  Clock : Clock
  Discrete-Time Integrator : DiscreteIntegrator  gainval=1  SampleTime=-1  ICPrevOutput=DiscIntNeverNeededParam  ICPrevScaledInput=DiscIntNeverNeededParam
  Divide : Product  Inputs=**
  Out1 : Outport
  wires:
  Discrete-Time Integrator/1 -> Out1/1
  In1/1 -> Abs/1
  Divide/1 -> Discrete-Time Integrator/1
  Abs/1 -> Divide/1
  Clock/1 -> Divide/2

== system APID/AREA 2/Performance Indices/ITSE ==
  In1 : Inport
  Clock : Clock
  Discrete-Time Integrator : DiscreteIntegrator  gainval=1  SampleTime=-1  ICPrevOutput=DiscIntNeverNeededParam  ICPrevScaledInput=DiscIntNeverNeededParam
  Divide : Product  Inputs=**
  Math Function : Math  Operator=square  SignedPower=on  SaturateOnIntegerOverflow=on
  Out1 : Outport
  wires:
  Discrete-Time Integrator/1 -> Out1/1
  In1/1 -> Math Function/1
  Divide/1 -> Discrete-Time Integrator/1
  Math Function/1 -> Divide/1
  Clock/1 -> Divide/2

== system APID/AREA 2/Performance Indices/Subsystem1 ==
  In1 : Inport
  Id_ref step : powerlib_extras/Control  Blocks/Timer  t=[0 1]  e=[0 1]
      settings: SourceProductBaseCode=PS
  Prod : Product  InputSameDT=on  SaturateOnIntegerOverflow=on  OutDataTypeStr=Inherit: Same as first input
  DP1 : Outport
  wires:
  Prod/1 -> DP1/1
  In1/1 -> Prod/1
  Id_ref step/1 -> Prod/2

== system APID/AREA 2/Performance Indices/Subsystem2 ==
  In1 : Inport
  Id_ref step : powerlib_extras/Control  Blocks/Timer  t=[0 1]  e=[0 1]
      settings: SourceProductBaseCode=PS
  Prod : Product  InputSameDT=on  SaturateOnIntegerOverflow=on  OutDataTypeStr=Inherit: Same as first input
  Out1 : Outport
  wires:
  Id_ref step/1 -> Prod/2
  In1/1 -> Prod/1
  Prod/1 -> Out1/1

== system APID/AREA 2/Performance Indices/Subsystem3 ==
  In1 : Inport
  Id_ref step : powerlib_extras/Control  Blocks/Timer  t=[0 1]  e=[0 1]
      settings: SourceProductBaseCode=PS
  Prod : Product  InputSameDT=on  SaturateOnIntegerOverflow=on  OutDataTypeStr=Inherit: Same as first input
  Out1 : Outport
  wires:
  Prod/1 -> Out1/1
  In1/1 -> Prod/1
  Id_ref step/1 -> Prod/2

== system APID/AREA 2/Performance Indices/Subsystem5 ==
  In1 : Inport
  Id_ref step : powerlib_extras/Control  Blocks/Timer  t=[0 1]  e=[0 1]
      settings: SourceProductBaseCode=PS
  Prod : Product  InputSameDT=on  SaturateOnIntegerOverflow=on  OutDataTypeStr=Inherit: Same as first input
  Out1 : Outport
  wires:
  Prod/1 -> Out1/1
  In1/1 -> Prod/1
  Id_ref step/1 -> Prod/2

== system APID/AREA 3/Adaptive PID3/Kd ==
  e : Inport
  Derivative : Derivative
  Product : Product  Inputs=3  RndMeth=Zero
  Sum2 : Sum
  Unit Delay : UnitDelay  InitialCondition=1.875  SampleTime=-1  HasFrameUpgradeWarning=on
  gamma : Constant  Value=gamma  SampleTime=0.001
  kd : Outport
  wires:
  Derivative/1 -> Product/2
  e/1 -> Product/3, Derivative/1
  gamma/1 -> Product/1
  Unit Delay/1 -> Sum2/1, kd/1
  Sum2/1 -> Unit Delay/1
  Product/1 -> Sum2/2

== system APID/AREA 3/Adaptive PID3/Ki ==
  e : Inport
  Math Function : Math  Operator=square  SignedPower=on  SaturateOnIntegerOverflow=on
  Product1 : Product  Inputs=3  RndMeth=Zero
  Sum1 : Sum
  Unit Delay1 : UnitDelay  InitialCondition=1.875  SampleTime=-1  HasFrameUpgradeWarning=on
  gamma1 : Constant  Value=gamma/2  SampleTime=0.001
  ki : Outport
  wires:
  gamma1/1 -> Product1/3
  Math Function/1 -> Product1/1
  Product1/1 -> Sum1/2
  e/1 -> Product1/2, Math Function/1
  Unit Delay1/1 -> ki/1, Sum1/1
  Sum1/1 -> Unit Delay1/1

== system APID/AREA 3/Adaptive PID3/Kp ==
  e : Inport
  Math Function : Math  Operator=square  SignedPower=on  SaturateOnIntegerOverflow=on
  Product : Product  RndMeth=Zero
  Sum2 : Sum
  Unit Delay : UnitDelay  InitialCondition=1.875  SampleTime=-1  HasFrameUpgradeWarning=on
  gamma : Constant  Value=gamma  SampleTime=0.001
  kp : Outport
  wires:
  Unit Delay/1 -> Sum2/1, kp/1
  Sum2/1 -> Unit Delay/1
  Product/1 -> Sum2/2
  gamma/1 -> Product/2
  Math Function/1 -> Product/1
  e/1 -> Math Function/1

== system APID/AREA 3/Performance Indices/IAE ==
  In1 : Inport
  Abs : Abs
  Discrete-Time Integrator : DiscreteIntegrator  gainval=1  SampleTime=-1  ICPrevOutput=DiscIntNeverNeededParam  ICPrevScaledInput=DiscIntNeverNeededParam
  Out1 : Outport
  wires:
  Abs/1 -> Discrete-Time Integrator/1
  Discrete-Time Integrator/1 -> Out1/1
  In1/1 -> Abs/1

== system APID/AREA 3/Performance Indices/ISE ==
  In1 : Inport
  Discrete-Time Integrator : DiscreteIntegrator  gainval=1  SampleTime=-1  ICPrevOutput=DiscIntNeverNeededParam  ICPrevScaledInput=DiscIntNeverNeededParam
  Math Function : Math  Operator=square  SignedPower=on  SaturateOnIntegerOverflow=on
  Out1 : Outport
  wires:
  In1/1 -> Math Function/1
  Discrete-Time Integrator/1 -> Out1/1
  Math Function/1 -> Discrete-Time Integrator/1

== system APID/AREA 3/Performance Indices/ITAE2 ==
  In1 : Inport
  Abs : Abs
  Clock : Clock
  Discrete-Time Integrator : DiscreteIntegrator  gainval=1  SampleTime=-1  ICPrevOutput=DiscIntNeverNeededParam  ICPrevScaledInput=DiscIntNeverNeededParam
  Divide : Product  Inputs=**
  Out1 : Outport
  wires:
  Discrete-Time Integrator/1 -> Out1/1
  In1/1 -> Abs/1
  Divide/1 -> Discrete-Time Integrator/1
  Abs/1 -> Divide/1
  Clock/1 -> Divide/2

== system APID/AREA 3/Performance Indices/ITSE ==
  In1 : Inport
  Clock : Clock
  Discrete-Time Integrator : DiscreteIntegrator  gainval=1  SampleTime=-1  ICPrevOutput=DiscIntNeverNeededParam  ICPrevScaledInput=DiscIntNeverNeededParam
  Divide : Product  Inputs=**
  Math Function : Math  Operator=square  SignedPower=on  SaturateOnIntegerOverflow=on
  Out1 : Outport
  wires:
  Discrete-Time Integrator/1 -> Out1/1
  In1/1 -> Math Function/1
  Divide/1 -> Discrete-Time Integrator/1
  Math Function/1 -> Divide/1
  Clock/1 -> Divide/2

== system APID/AREA 3/Performance Indices/Subsystem1 ==
  In1 : Inport
  Id_ref step : powerlib_extras/Control  Blocks/Timer  t=[0 1]  e=[0 1]
      settings: SourceProductBaseCode=PS
  Prod : Product  InputSameDT=on  SaturateOnIntegerOverflow=on  OutDataTypeStr=Inherit: Same as first input
  Out1 : Outport
  wires:
  Id_ref step/1 -> Prod/2
  In1/1 -> Prod/1
  Prod/1 -> Out1/1

== system APID/AREA 3/Performance Indices/Subsystem2 ==
  In1 : Inport
  Id_ref step : powerlib_extras/Control  Blocks/Timer  t=[0 1]  e=[0 1]
      settings: SourceProductBaseCode=PS
  Prod : Product  InputSameDT=on  SaturateOnIntegerOverflow=on  OutDataTypeStr=Inherit: Same as first input
  DP1 : Outport
  wires:
  Prod/1 -> DP1/1
  In1/1 -> Prod/1
  Id_ref step/1 -> Prod/2

== system APID/AREA 3/Performance Indices/Subsystem3 ==
  In1 : Inport
  Id_ref step : powerlib_extras/Control  Blocks/Timer  t=[0 1]  e=[0 1]
      settings: SourceProductBaseCode=PS
  Prod : Product  InputSameDT=on  SaturateOnIntegerOverflow=on  OutDataTypeStr=Inherit: Same as first input
  Out1 : Outport
  wires:
  Prod/1 -> Out1/1
  In1/1 -> Prod/1
  Id_ref step/1 -> Prod/2

== system APID/AREA 3/Performance Indices/Subsystem5 ==
  In1 : Inport
  Id_ref step : powerlib_extras/Control  Blocks/Timer  t=[0 1]  e=[0 1]
      settings: SourceProductBaseCode=PS
  Prod : Product  InputSameDT=on  SaturateOnIntegerOverflow=on  OutDataTypeStr=Inherit: Same as first input
  Out1 : Outport
  wires:
  Prod/1 -> Out1/1
  In1/1 -> Prod/1
  Id_ref step/1 -> Prod/2

== system APID/AREA 4/Adaptive PID3/Kd ==
  e : Inport
  Derivative : Derivative
  Product : Product  Inputs=3  RndMeth=Zero
  Sum2 : Sum
  Unit Delay : UnitDelay  InitialCondition=1.875  SampleTime=-1  HasFrameUpgradeWarning=on
  gamma : Constant  Value=gamma  SampleTime=0.001
  kd : Outport
  wires:
  Derivative/1 -> Product/2
  e/1 -> Product/3, Derivative/1
  gamma/1 -> Product/1
  Unit Delay/1 -> Sum2/1, kd/1
  Sum2/1 -> Unit Delay/1
  Product/1 -> Sum2/2

== system APID/AREA 4/Adaptive PID3/Ki ==
  e : Inport
  Math Function : Math  Operator=square  SignedPower=on  SaturateOnIntegerOverflow=on
  Product1 : Product  Inputs=3  RndMeth=Zero
  Sum1 : Sum
  Unit Delay1 : UnitDelay  InitialCondition=1.875  SampleTime=-1  HasFrameUpgradeWarning=on
  gamma1 : Constant  Value=gamma/2  SampleTime=0.001
  ki : Outport
  wires:
  gamma1/1 -> Product1/3
  Math Function/1 -> Product1/1
  Product1/1 -> Sum1/2
  e/1 -> Product1/2, Math Function/1
  Unit Delay1/1 -> ki/1, Sum1/1
  Sum1/1 -> Unit Delay1/1
